simulink model "AnimateActorWithKinematics"  (R2024a)
settings: Solver=VariableStepAuto  StartTime=0.0  StopTime=10.0  RelTol=1e-3
libraries: sim3dlib x3
settings Model: Creator=Miko  LastModifiedBy=Miko

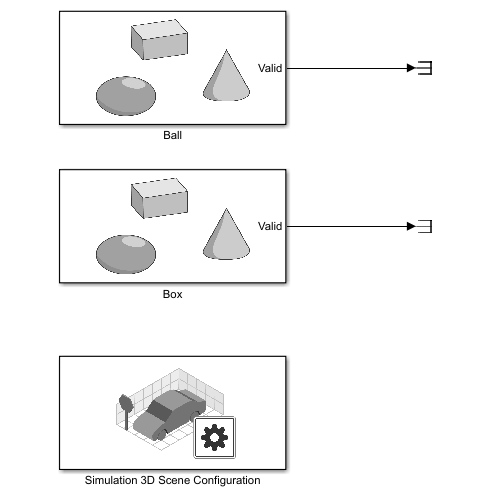
[thumbnail: Simulink's stored preview of the top-level diagram]
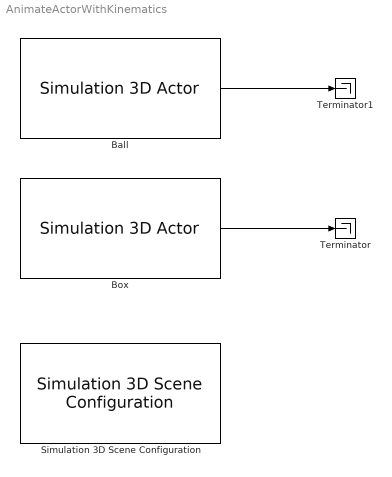
== system AnimateActorWithKinematics ==
  Ball : sim3dlib/Simulation 3D Actor  Priority=1  ActorName=Ball  ParentName=Scene Origin  Operation=Create at setup  InitScriptText=|  SampleTime=-1  Translation=[1 -2 1]  Rotation=single([0 0 0])  Scale=single([1 1 1])  aMode=5  ActorTag=Ball  ActorType=Sim3dActor  ID=C
      | Actor.createShape('sphere', [0.5, 0.5, 0.5]); % 球體半徑
      | Actor.Mobility = sim3d.utils.MobilityTypes.Movable; % 球體移動設定
      | Actor.LinearVelocity = [0, 0.5, 0];
      | Actor.Color = [0, 1, 1]; % 顏色(RGB參數)
      | % Actor.Gravity = true; % 引力
      | % Actor.Physics = true; % 外觀
      | % Actor.Shadows = false; % 陰影(無)
  Box : sim3dlib/Simulation 3D Actor  Priority=1  ActorName=Box  ParentName=Scene Origin  Operation=Create at setup  InitScriptText=|  SampleTime=-1  Translation=single([1 0 -1])  Rotation=single([0 0 0])  Scale=single([1 1 1])  aMode=5  ActorTag=Box  ActorType=Sim3dActor  ID=C
      | Actor.createShape('box', [0.5 0.5 0.5]);
      | Actor.Mobility = sim3d.utils.MobilityTypes.Movable;
      | Actor.AngularVelocity = [0, 0, pi/4];
      | Actor.Color = [1, 0, 1];
  Simulation 3D Scene Configuration : sim3dlib/Simulation 3D Scene Configuration  Priority=0  ProjectFormat=Default Scenes  SceneDesc=Empty scene  ProjectName=C:\Program Files\MATLAB\R2024a\toolbox\shared\sim3d_projects\automotive_project_windows\UE\WindowsNoEditor\VehicleSimulation.exe  ScenePath=/Game/Maps/HwStrght  EnableOpenDRIVE=off  vehTagList={'Ball';'Box';'Custom';'Scene Origin'}  vehTag=Scene Origin  FreeCameraInitialTranslation=[0, 0, 0]  FreeCameraDefaultInitialTranslation=[-6, 0, 2]  FreeCameraInitialRotation=[0, 0, 0]  FreeCameraDefaultInitialRotation=[0, -15, 0]  OpVisEn=off  Ts=.02  EnableWindow=on  EnableRemoteAccess=off  EnableWeather=off  SunAzimuth=90  SunAltitude=40.0  EnableGeospatialSun=off  Latitude=0  Longitude=0  Date=2023-01-01  Time=10:30:00  GeoTimeZone=-5.0  SunDaylightSaving=off  wind=1  clouds=10  EnableVolumetricClouds=off  CloudCoverage=0  CloudAltitude=6  fog=0  rain=0  RaindropsEffect=off  SnowDensity=0  EnableGeospatial=off  UseTrueOrigin=off  OriginHeight=200  OriginLatitude=40.744652  OriginLongitude=-73.988864  MapStyle=Aerial  AdditionalAssetIDs=[]  UseAdvancedSunSky=off  SolarTime=11  TimeZone=-5  Day=21  Month=9  Year=2022  UseDaylightSavingTime=on  DSTStartDay=10  DSTStartMonth=3  DSTEndDay=3  DSTEndMonth=11  DSTSwitchHour=2  sensorTag=MainCamera1  sensorId=1  sensorName=MainCamera1  mountLoc=Origin  offsetFlag=off  tmountOffset=[0, 0, 0]  rmountOffset=[0, 0, 0]  HorizontalResolution=1280  VerticalResolution=720  HorizontalFOV=60  mountPoint=[0 0 0]  mountOrientation=[0 0 0]  aMode=5  ID=1  GeoTrigger=Inactive
      settings: LibrarySourceBlock=sl3dlib/Simulation 3D/Environment/Simulation 3D Scene Configuration
  Terminator : Terminator
  Terminator1 : Terminator
  wires:
  Box/1 -> Terminator/1
  Ball/1 -> Terminator1/1
